simulink model "demo_Stack_IronAir"  (R2025b)
settings: Solver=ode15s  StartTime=0.0  StopTime=1800  RelTol=1e-3
libraries: lib_IronAir x2
settings Model: Creator=admin  LastModifiedBy=admin

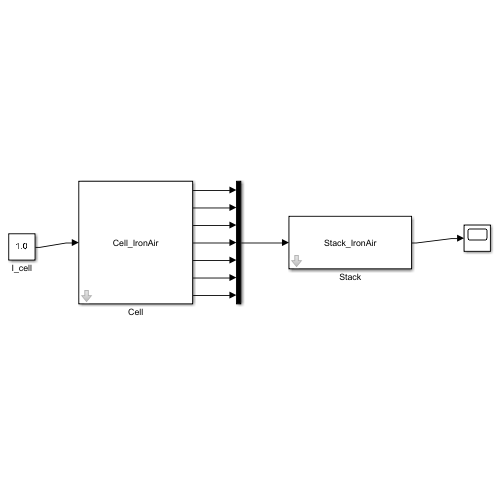
[thumbnail: Simulink's stored preview of the top-level diagram]
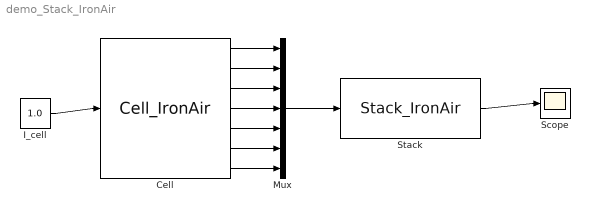
== system demo_Stack_IronAir ==
  Cell : lib_IronAir/Cell_IronAir
  I_cell : Constant  Value=1.0
  Mux : Mux  Inputs=7
  Scope : Scope
  Stack : lib_IronAir/Stack_IronAir
  wires:
  I_cell/1 -> Cell/1
  Cell/1 -> Mux/1
  Cell/2 -> Mux/2
  Cell/3 -> Mux/3
  Cell/4 -> Mux/4
  Cell/5 -> Mux/5
  Cell/6 -> Mux/6
  Cell/7 -> Mux/7
  Mux/1 -> Stack/1
  Stack/1 -> Scope/1
